simulink model "circuitbreaker_1"  (Simulink 7.4)
settings: Solver=ode23t  StartTime=0.0  StopTime=10.0  MaxStep=.02  RelTol=1e-3
undefined symbols (not defined in the file or in its folder): sigbuilder_block
libraries: powerlib x7, simulink x1, simulink_extras x1
settings Model: Creator=dbenson  LastModifiedBy=Dick
settings DataIOCC: SignalLoggingName=sigsOut
settings OptimizationCC: InitFltsAndDblsToZero=on
settings DebuggingCC: SaveWithParameterizedLinksMsg=none  SignalResolutionControl=TryResolveAllWithWarning  SolverPrmCheckMsg=none  MultiTaskDSMMsg=warning  MultiTaskCondExecSysMsg=none  StrictBusMsg=None
settings HardwareCC: TargetUnknown=on
settings RTWCC: IncludeERTFirstTime=on

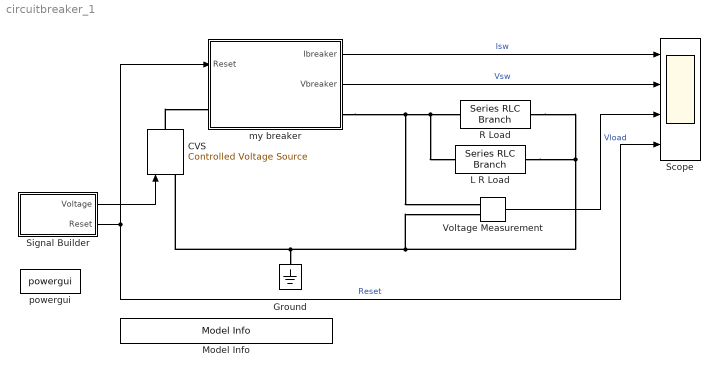
== system circuitbreaker_1 ==
  CVS : powerlib/Electrical Sources/Controlled Voltage Source  Description=source block  DialogController=POWERSYS.PowerSysDialog  SystemSampleTime=-1  Initialize=off  Source_Type=AC  Amplitude=0  Phase=0  Frequency=0  Measurements=None
      settings: AttributesFormatString=\n
  Ground : powerlib/Elements/Ground  DialogController=POWERSYS.PowerSysDialog  PhysicalDomain=powersysdomain  SubClassName=unknown  LeftPortType=p1  RightPortType=p1  LConnTagsString=a
  L R Load : powerlib/Elements/Series RLC Branch  DialogController=POWERSYS.PowerSysDialog  PhysicalDomain=powersysdomain  SubClassName=unknown  LeftPortType=p1  RightPortType=p1  LConnTagsString=__new0  RConnTagsString=__new0  BranchType=RL  Resistance=1.3333333  Inductance=10e-3  SetiL0=off  InitialCurrent=0  Capacitance=1.0  Setx0=off  InitialVoltage=0  Measurements=None
  Model Info : simulink/Model-Wide Utilities/Model Info  SystemSampleTime=-1  InitialBlockCM=None  BlockCM=None  Frame=on  DisplayStringWithTags=Copywrite 2005-2010 The MathWorks, Inc.  HorizontalTextAlignment=Center  LeftAlignmentValue=0.5  SourceBlockDiagram=circuitbreaker_1  TagMaxNumber=20
  R Load : powerlib/Elements/Series RLC Branch  DialogController=POWERSYS.PowerSysDialog  PhysicalDomain=powersysdomain  SubClassName=unknown  LeftPortType=p1  RightPortType=p1  LConnTagsString=__new0  RConnTagsString=__new0  BranchType=R  Resistance=4  Inductance=1.0  SetiL0=off  InitialCurrent=0  Capacitance=1.0  Setx0=off  InitialVoltage=0  Measurements=None
  Scope : Scope  NumInputPorts=4
      settings: TimeRange=10  YMin=0~0~-100~0  YMax=20~100~100~1
  Signal Builder : Subsystem  Tag=STV Subsys  LoadFcn=sigbuilder_block('load');  StartFcn=sigbuilder_block('start');  StopFcn=sigbuilder_block('stop');  ClipboardFcn=sigbuilder_block('clipboard');  mask(Sigbuilder block){}
      mask help: Sigbuilder GUI
      mask init:
      | if ~strcmp(get_param(bdroot,'SimulationStatus'),'stopped') tuvar = sigbuilder_block('maskInit'); end
      settings: CopyFcn=sigbuilder_block('copy');  DeleteFcn=sigbuilder_block('delete');  ModelCloseFcn=sigbuilder_block('modelClose');  PreSaveFcn=sigbuilder_block('preSave');  NameChangeFcn=sigbuilder_block('namechange');  OpenFcn=sigbuilder_block('open',[44.25 356.25 526.5 286.5 ]);  CloseFcn=sigbuilder_block('close');
      mask Display: plot(0,0,100,100,[10,10,40,40,10],[80,20,20,80,80],[40,10],[50,50], [40,27,10],[65,72,56],[40,25,25,10],[28,28,43,43]);
  Voltage Measurement : powerlib/Measurements/Voltage Measurement  Tag=PoWeRsYsTeMmEaSuReMeNt  DialogController=POWERSYS.PowerSysDialog  SystemSampleTime=-1  PhasorSimulation=off  OutputType=Magnitude  PSBequivalent=0
  my breaker : Subsystem  mask{Iset=10, Tau=.1}
      mask prompts: Iset "Current Rating (Amps)"; Tau "Mechanical Time Constant (Sec)"
  powergui : powerlib/powergui  SystemSampleTime=-1  SimulationMode=Continuous  SampleTime=50e-6  frequency=60  SPID=off  DisableSnubberDevices=off  DisableRonSwitches=off  DisableVfSwitches=off  SwTol=0  Interpol=off  frequencyindice=0  echomessages=off  HookPort=off  DisplayEquations=off  FunctionMessages=off  EnableUseOfTLC=off  x0status=blocks  RestoreLinks=warning  Frange=[0:2:500]  Ylog=off  Xlog=on  ShowGrid=off  save=off  variable=ZData  ZoomFFT=on  StartTime=0.0  cycles=1  DisplayStyle=1  fundamental=60  FreqAxis=off  MaxFrequency=1000  frequencyindicesteady=1  RmsSteady=1  display=off  Ts=0  methode=off
  wires:
  Signal Builder/1(Voltage) -> CVS/1
  Signal Builder/2(Reset) -> my breaker/1(Reset), Scope/4  "Reset"
  Voltage Measurement/1 -> Scope/3  "Vload"
  my breaker/1(Ibreaker) -> Scope/1  "Isw"
  my breaker/2(Vbreaker) -> Scope/2  "Vsw"
  connections:
  R Load/RConn1 -- Ground/LConn1 -- CVS/LConn1 -- Voltage Measurement/LConn2 -- L R Load/RConn1
  CVS/RConn1 -- my breaker/LConn1
  my breaker/RConn1 -- Voltage Measurement/LConn1 -- R Load/LConn1 -- L R Load/LConn1

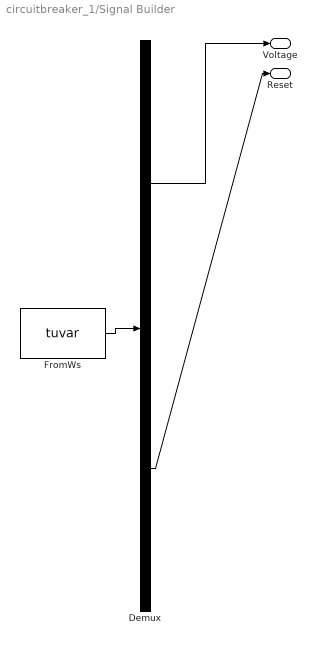
== system circuitbreaker_1/Signal Builder ==
  Demux : Demux  Tag=STV Demux  Outputs=2
  FromWs : FromWorkspace  Tag=STV FromWs  VariableName=tuvar  SampleTime=0  SigBuilderData=DataTag0  VnvData=DataTag1
      SigBuilderData=|
      | channels(1).label = 'Voltage'
      | channels(1).allXData = {[0 1 1 1.16 1.16 10]}
      | channels(1).allYData = {[0 0 19.6 19.6 6.8 15.2]}
      | channels(2).label = 'Reset'
      | channels(2).allXData = {[0 3.62 3.62 3.66 3.66 10]}
      | channels(2).allYData = {[0 0 1 1 0 0]}
      | dataSet.timeRange = [0 10]
      | dataSet.name = 'Group 1'
  Voltage : Outport  Tag=STV Outport
  Reset : Outport  Tag=STV Outport  Port=2
  wires:
  Demux/1 -> Voltage/1
  FromWs/1 -> Demux/1
  Demux/2 -> Reset/1

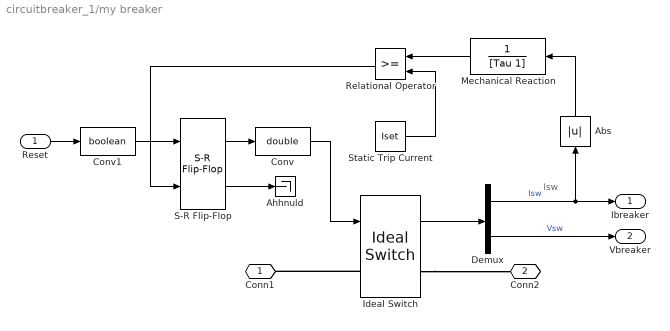
== system circuitbreaker_1/my breaker ==
  note: Isw
  Reset : Inport  OutDataType=sfix(16)  OutScaling=2^0
  Abs : Abs  SaturateOnIntegerOverflow=on
  Ahhnuld : Terminator
  Conv : DataTypeConversion  OutDataTypeMode=double  OutDataTypeStr=double  SaturateOnIntegerOverflow=on  RndMeth=Zero
  Conv1 : DataTypeConversion  OutDataTypeMode=boolean  OutDataTypeStr=boolean  SaturateOnIntegerOverflow=on  RndMeth=Zero
  Demux : Demux  Outputs=2
  Ideal Switch : powerlib/Power Electronics/Ideal Switch  DialogController=POWERSYS.PowerSysDialog  SystemSampleTime=-1  Ron=0.001  Lon=0  IC=1  Rs=0  Cs=0  Measurements=on
      settings: AttributesFormatString=\n
  Mechanical Reaction : TransferFcn  Denominator=[Tau 1]
  Relational Operator : RelationalOperator
  S-R Flip-Flop : simulink_extras/Flip Flops/S-R Flip-Flop  SystemSampleTime=-1  initial_condition=1
  "Static Trip Current " : Constant  Value=Iset  OutDataType=sfix(16)  OutScaling=2^0
  Conn1 : PMIOPort  Port=1  Side=Left
  Conn2 : PMIOPort  Port=2  Side=Right
  Ibreaker : Outport
  Vbreaker : Outport  Port=2
  wires:
  Ideal Switch/1 -> Demux/1
  Demux/1 -> Ibreaker/1, Abs/1  "Isw"
  Mechanical Reaction/1 -> Relational Operator/1
  "Static Trip Current "/1 -> Relational Operator/2
  S-R Flip-Flop/1 -> Conv/1
  Conv/1 -> Ideal Switch/1
  Demux/2 -> Vbreaker/1  "Vsw"
  Reset/1 -> Conv1/1
  Conv1/1 -> S-R Flip-Flop/1
  S-R Flip-Flop/2 -> Ahhnuld/1
  Relational Operator/1 -> S-R Flip-Flop/2
  Abs/1 -> Mechanical Reaction/1
  connections:
  Ideal Switch/LConn1 -- Conn1/RConn1
  Ideal Switch/RConn1 -- Conn2/RConn1
